simulink library "ConversionsLibrary"  (R2016b)
settings: Solver=VariableStepAuto  StartTime=0.0  StopTime=10.0  RelTol=1e-3
settings Model: Creator=Nathan  LastModifiedBy=march

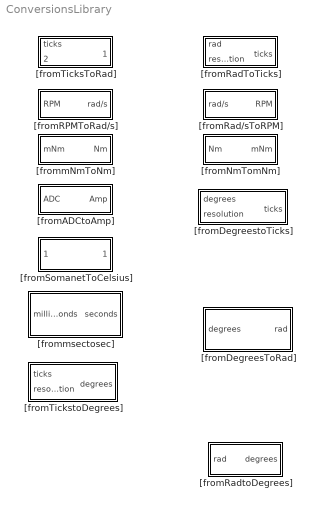
== system ConversionsLibrary ==
  "[fromADCtoAmp]" : Subsystem
  "[fromDegreesToRad]" : Subsystem
  "[fromDegreestoTicks]" : Subsystem
  "[fromNmTomNm]" : Subsystem
  "[fromRPMToRad/s]" : Subsystem
  "[fromRad/sToRPM]" : Subsystem
  "[fromRadToTicks]" : Subsystem
  "[fromRadtoDegrees]" : Subsystem
  "[fromSomanetToCelsius]" : Subsystem
  "[fromTicksToRad]" : Subsystem
  "[fromTickstoDegrees]" : Subsystem
  "[frommNmToNm]" : Subsystem
  "[frommsectosec]" : Subsystem

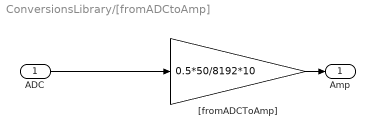
== system ConversionsLibrary/[fromADCtoAmp] ==
  ADC : Inport
  "[fromADCToAmp]" : Gain  Gain=0.5*50/8192*10
  Amp : Outport
  wires:
  "[fromADCToAmp]"/1 -> Amp/1
  ADC/1 -> "[fromADCToAmp]"/1

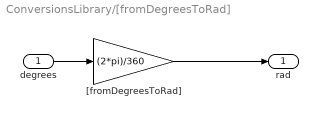
== system ConversionsLibrary/[fromDegreesToRad] ==
  degrees : Inport
  "[fromDegreesToRad]" : Gain  Gain=(2*pi)/360
  rad : Outport
  wires:
  "[fromDegreesToRad]"/1 -> rad/1
  degrees/1 -> "[fromDegreesToRad]"/1

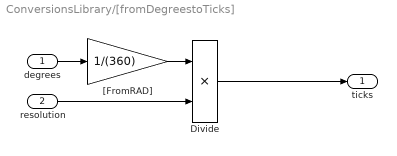
== system ConversionsLibrary/[fromDegreestoTicks] ==
  degrees : Inport
  resolution : Inport  Port=2
  Divide : Product  Inputs=**
  "[FromRAD]" : Gain  Gain=1/(360)
  ticks : Outport
  wires:
  Divide/1 -> ticks/1
  degrees/1 -> "[FromRAD]"/1
  "[FromRAD]"/1 -> Divide/1
  resolution/1 -> Divide/2

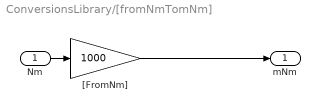
== system ConversionsLibrary/[fromNmTomNm] ==
  Nm : Inport
  "[FromNm]" : Gain  Gain=1000
  mNm : Outport
  wires:
  Nm/1 -> "[FromNm]"/1
  "[FromNm]"/1 -> mNm/1

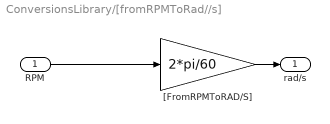
== system ConversionsLibrary/[fromRPMToRad//s] ==
  RPM : Inport
  "[FromRPMToRAD/S]" : Gain  Gain=2*pi/60
  rad/s : Outport
  wires:
  "[FromRPMToRAD/S]"/1 -> rad/s/1
  RPM/1 -> "[FromRPMToRAD/S]"/1

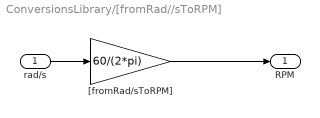
== system ConversionsLibrary/[fromRad//sToRPM] ==
  rad/s : Inport
  "[fromRad/sToRPM]" : Gain  Gain=60/(2*pi)
  RPM : Outport
  wires:
  rad/s/1 -> "[fromRad/sToRPM]"/1
  "[fromRad/sToRPM]"/1 -> RPM/1

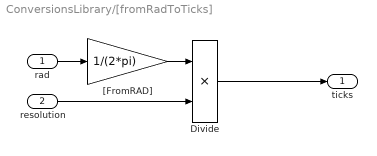
== system ConversionsLibrary/[fromRadToTicks] ==
  rad : Inport
  resolution : Inport  Port=2
  Divide : Product  Inputs=**
  "[FromRAD]" : Gain  Gain=1/(2*pi)
  ticks : Outport
  wires:
  rad/1 -> "[FromRAD]"/1
  "[FromRAD]"/1 -> Divide/1
  resolution/1 -> Divide/2
  Divide/1 -> ticks/1

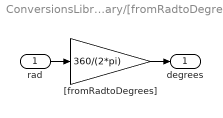
== system ConversionsLibrary/[fromRadtoDegrees] ==
  rad : Inport
  "[fromRadtoDegrees]" : Gain  Gain=360/(2*pi)
  degrees : Outport
  wires:
  "[fromRadtoDegrees]"/1 -> degrees/1
  rad/1 -> "[fromRadtoDegrees]"/1

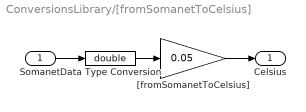
== system ConversionsLibrary/[fromSomanetToCelsius] ==
  Somanet : Inport
  Data Type Conversion : DataTypeConversion  OutDataTypeStr=double
  "[fromSomanetToCelsius]" : Gain  Gain=0.05
  Celsius : Outport
  wires:
  Somanet/1 -> Data Type Conversion/1
  "[fromSomanetToCelsius]"/1 -> Celsius/1
  Data Type Conversion/1 -> "[fromSomanetToCelsius]"/1

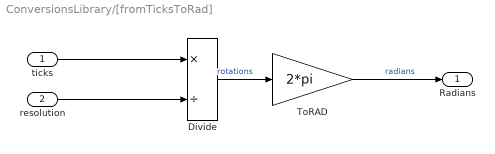
== system ConversionsLibrary/[fromTicksToRad] ==
  ticks : Inport
  resolution : Inport  Port=2
  Divide : Product  Inputs=*/
  ToRAD : Gain  Gain=2*pi
  Radians : Outport
  wires:
  ToRAD/1 -> Radians/1  "radians"
  resolution/1 -> Divide/2
  Divide/1 -> ToRAD/1  "rotations"
  ticks/1 -> Divide/1

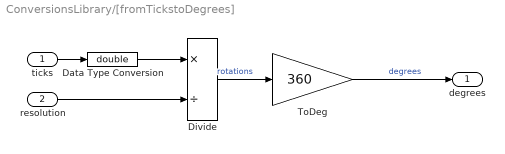
== system ConversionsLibrary/[fromTickstoDegrees] ==
  ticks : Inport
  resolution : Inport  Port=2
  Data Type Conversion : DataTypeConversion  OutDataTypeStr=double
  Divide : Product  Inputs=*/
  ToDeg : Gain  Gain=360
  degrees : Outport
  wires:
  ToDeg/1 -> degrees/1  "degrees"
  ticks/1 -> Data Type Conversion/1
  resolution/1 -> Divide/2
  Divide/1 -> ToDeg/1  "rotations"
  Data Type Conversion/1 -> Divide/1

== system ConversionsLibrary/[frommNmToNm] ==
  mNm : Inport
  "[ToNm]" : Gain  Gain=1/1000
  Nm : Outport
  wires:
  "[ToNm]"/1 -> Nm/1
  mNm/1 -> "[ToNm]"/1

== system ConversionsLibrary/[frommsectosec] ==
  milliseconds : Inport
  Gain : Gain  Gain=1/1000
  seconds : Outport
  wires:
  Gain/1 -> seconds/1
  milliseconds/1 -> Gain/1
